simulink model "humanoidRobotIcub"  (Simulink 9.2)
settings: Solver=FixedStepAuto  StartTime=0.0  StopTime=10.0  FixedStep=0.001  RelTol=1e-3
undefined symbols (not defined in the file): DESIRED_TRAJECTORY_IS_FIXED, dq_max, dq_min, k1, k2, k3, q_des_amp, q_des_bias, q_des_freq, q_des_phase, q_max, q_min
libraries: WBToolboxLibrary x9
settings Model: Creator=venus.pasandi  LastModifiedBy=venus.pasandi
settings DataIOCC: LimitDataPoints=off  SaveFormat=Dataset  SignalLoggingSaveFormat=Dataset
settings OptimizationCC: LifeSpan=auto
settings DebuggingCC: UnderspecifiedInitializationDetection=Simplified  MergeDetectMultiDrivingBlocksExec=error  FcnCallInpInsideContextMsg=error  StateNameClashWarn=none  SFUnexpectedBacktrackingDiag=error  SFNoUnconditionalDefaultTransitionDiag=error  SFExecutionAtInitializationDiag=warning
settings HardwareCC: ProdBitPerPointer=64  ProdBitPerSizeT=64  ProdBitPerPtrDiffT=64  ProdLargestAtomicFloat=Float  ProdIntDivRoundTo=Zero  ProdEndianess=LittleEndian  ProdWordSize=64  ProdHWDeviceType=Intel->x86-64 (Windows64)
settings ModelReferenceCC: PropagateSignalLabelsOutOfModel=on
settings SFSimCC: SimUseLocalCustomCode=on
settings RTWCC: RTWUseLocalCustomCode=on
settings CodeAppCC: StateflowObjectComments=off
settings GRTTargetCC: TargetLangStandard=C99 (ISO)  GeneratePreprocessorConditionals=Use local settings  CombineOutputUpdateFcns=on  GRTInterface=off
settings ConfigComp: CovMetricSettings=dwe  CovHtmlReporting=off  CovSaveCumulativeToWorkspaceVar=off  CovSaveSingleToWorkspaceVar=off  CovExternalEMLEnable=on

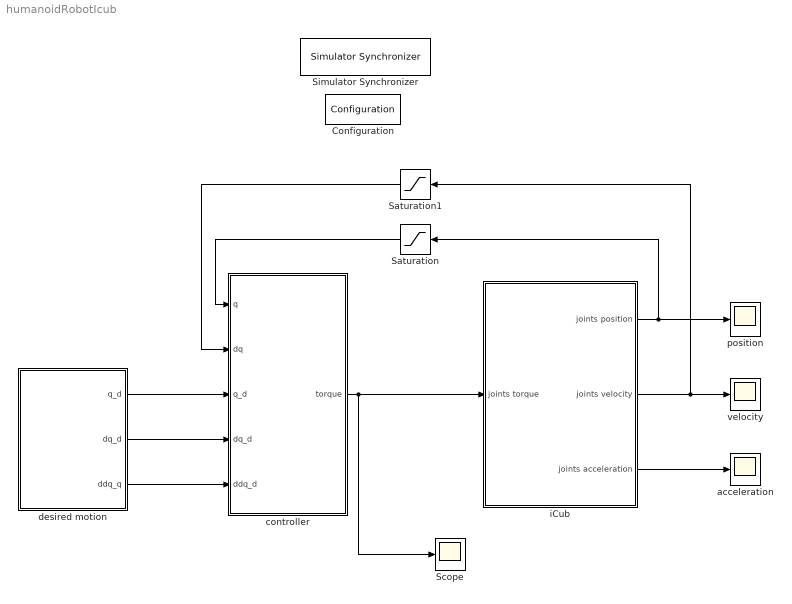
== system humanoidRobotIcub ==
  Configuration : WBToolboxLibrary/Utilities/Configuration  ConfigSource=Mask  ConfigObject='WBTConfigRobot'  RobotName='icubSim'  UrdfFile='model.urdf'  ControlledJoints={'r_hip_pitch', 'r_hip_roll', 'r_knee'}  ControlBoardsNames={'right_leg'}  LocalName='WBT'  GravityVector=[0,0,-9.81]
      settings: SourceProductName=WholeBodyToolbox
  Saturation : Saturate  UpperLimit=q_max-0.001  LowerLimit=q_min+0.001
  Saturation1 : Saturate  UpperLimit=dq_max-0.001  LowerLimit=dq_min+0.001
  Scope : Scope
  Simulator Synchronizer : WBToolboxLibrary/Utilities/Simulator Synchronizer  period=0.001  serverPortName='/clock/rpc'  clientPortName='/WBT_synchronizer/rpc:o'
      settings: SourceProductName=WholeBodyToolbox
  acceleration : Scope
  controller : Subsystem
  desired motion : Subsystem
  iCub : Subsystem
  position : Scope
  velocity : Scope
  wires:
  iCub/1(joints position) -> Saturation/1, position/1
  iCub/2(joints velocity) -> Saturation1/1, velocity/1
  iCub/3(joints acceleration) -> acceleration/1
  controller/1(torque) -> Scope/1, iCub/1(joints torque)
  desired motion/1(q_d) -> controller/3(q_d)
  desired motion/2(dq_d) -> controller/4(dq_d)
  desired motion/3(ddq_q) -> controller/5(ddq_d)
  Saturation/1 -> controller/1(q)
  Saturation1/1 -> controller/2(dq)

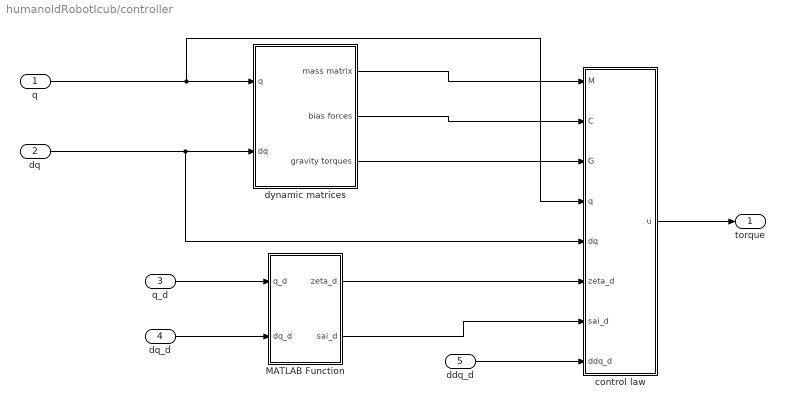
== system humanoidRobotIcub/controller ==
  q : Inport
  dq : Inport  Port=2
  q_d : Inport  Port=3
  dq_d : Inport  Port=4
  ddq_d : Inport  Port=5
  MATLAB Function : MATLAB Function  TreatAsAtomicUnit=on
  control law : MATLAB Function  TreatAsAtomicUnit=on
  dynamic matrices : Subsystem
  torque : Outport  VectorParamsAs1DForOutWhenUnconnected=on
  wires:
  dq_d/1 -> MATLAB Function/2(dq_d)
  q_d/1 -> MATLAB Function/1(q_d)
  MATLAB Function/2(sai_d) -> control law/7(sai_d)
  MATLAB Function/1(zeta_d) -> control law/6(zeta_d)
  control law/1(u) -> torque/1
  ddq_d/1 -> control law/8(ddq_d)
  dynamic matrices/3(gravity torques) -> control law/3(G)
  dynamic matrices/2(bias forces) -> control law/2(C)
  dynamic matrices/1(mass matrix) -> control law/1(M)
  dq/1 -> dynamic matrices/2(dq), control law/5(dq)
  q/1 -> control law/4(q), dynamic matrices/1(q)

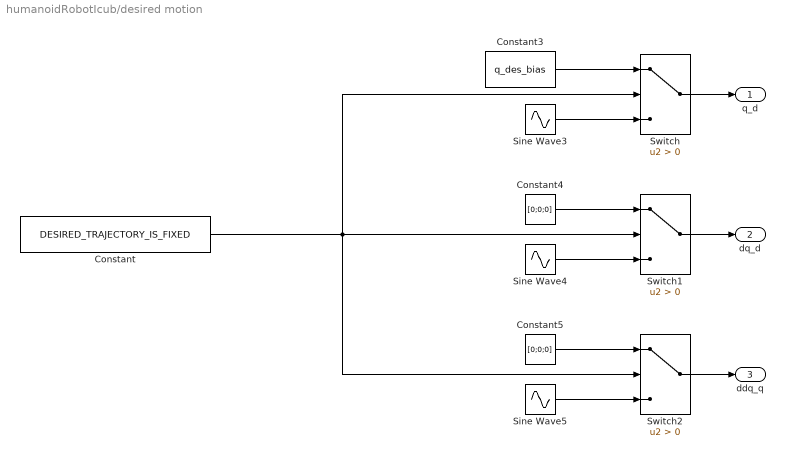
== system humanoidRobotIcub/desired motion ==
  Constant : Constant  Value=DESIRED_TRAJECTORY_IS_FIXED
  Constant3 : Constant  Value=q_des_bias
  Constant4 : Constant  Value=[0;0;0]
  Constant5 : Constant  Value=[0;0;0]
  Sine Wave3 : Sin  Amplitude=q_des_amp  Bias=q_des_bias  Frequency=q_des_freq  Phase=q_des_phase  SampleTime=0
  Sine Wave4 : Sin  Amplitude=q_des_amp .* q_des_freq  Bias=[0;0;0]  Frequency=q_des_freq  Phase=q_des_phase+pi/2  SampleTime=0
  Sine Wave5 : Sin  Amplitude=-q_des_amp .* (q_des_freq .^ 2)  Bias=[0;0;0]  Frequency=q_des_freq  Phase=q_des_phase  SampleTime=0
  Switch : Switch  Criteria=u2 > Threshold
  Switch1 : Switch  Criteria=u2 > Threshold
  Switch2 : Switch  Criteria=u2 > Threshold
  q_d : Outport  VectorParamsAs1DForOutWhenUnconnected=on
  dq_d : Outport  Port=2  VectorParamsAs1DForOutWhenUnconnected=on
  ddq_q : Outport  Port=3  VectorParamsAs1DForOutWhenUnconnected=on
  wires:
  Sine Wave5/1 -> Switch2/3
  Constant5/1 -> Switch2/1
  Constant4/1 -> Switch1/1
  Sine Wave4/1 -> Switch1/3
  Sine Wave3/1 -> Switch/3
  Constant3/1 -> Switch/1
  Constant/1 -> Switch/2, Switch2/2, Switch1/2
  Switch2/1 -> ddq_q/1
  Switch1/1 -> dq_d/1
  Switch/1 -> q_d/1

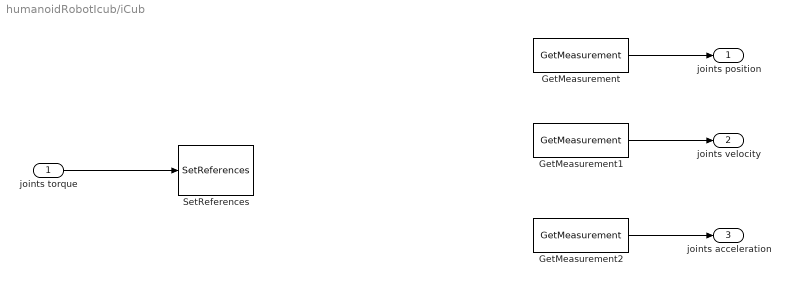
== system humanoidRobotIcub/iCub ==
  joints torque : Inport
  GetMeasurement : WBToolboxLibrary/States/GetMeasurement  measuredType=Joints Position
      settings: SourceProductName=WholeBodyToolbox
  GetMeasurement1 : WBToolboxLibrary/States/GetMeasurement  measuredType=Joints Velocity
      settings: SourceProductName=WholeBodyToolbox
  GetMeasurement2 : WBToolboxLibrary/States/GetMeasurement  measuredType=Joints Acceleration
      settings: SourceProductName=WholeBodyToolbox
  SetReferences : WBToolboxLibrary/Actuators/SetReferences  controlType=Torque  refSpeed=10*(pi/180)  refAcceleration=1000000*(pi/180)
      settings: SourceProductName=WholeBodyToolbox
  joints position : Outport
  joints velocity : Outport  Port=2
  joints acceleration : Outport  Port=3
  wires:
  GetMeasurement/1 -> joints position/1
  GetMeasurement1/1 -> joints velocity/1
  GetMeasurement2/1 -> joints acceleration/1
  joints torque/1 -> SetReferences/1

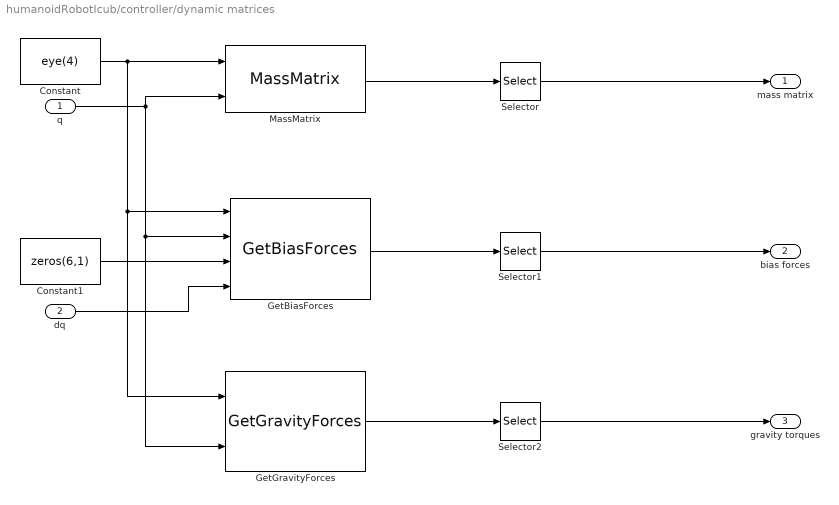
== system humanoidRobotIcub/controller/dynamic matrices ==
  q : Inport
  dq : Inport  Port=2
  Constant : Constant  Value=eye(4)
  Constant1 : Constant  Value=zeros(6,1)
  GetBiasForces : WBToolboxLibrary/Model/Dynamics/GetBiasForces
      settings: SourceProductName=WholeBodyToolbox
  GetGravityForces : WBToolboxLibrary/Model/Dynamics/GetGravityForces
      settings: SourceProductName=WholeBodyToolbox
  MassMatrix : WBToolboxLibrary/Model/Dynamics/MassMatrix
      settings: SourceProductName=WholeBodyToolbox
  Selector : Selector  NumberOfDimensions=2  InputPortWidth=3  IndexOptions=Index vector (dialog),Index vector (dialog)  Indices=[7:9],[7:9]  OutputSizes=1,1
  Selector1 : Selector  InputPortWidth=9  IndexOptions=Index vector (dialog)  Indices=[7:9]  OutputSizes=1
  Selector2 : Selector  InputPortWidth=9  IndexOptions=Index vector (dialog)  Indices=[7:9]  OutputSizes=1
  mass matrix : Outport
  bias forces : Outport  Port=2
  gravity torques : Outport  Port=3
  wires:
  Selector2/1 -> gravity torques/1
  Selector1/1 -> bias forces/1
  Selector/1 -> mass matrix/1
  dq/1 -> GetBiasForces/4
  Constant1/1 -> GetBiasForces/3
  GetBiasForces/1 -> Selector1/1
  GetGravityForces/1 -> Selector2/1
  MassMatrix/1 -> Selector/1
  q/1 -> MassMatrix/2, GetBiasForces/2, GetGravityForces/2
  Constant/1 -> MassMatrix/1, GetGravityForces/1, GetBiasForces/1

== matlab function controller/control law ==
  data: M input double; C input double; G input double; q input double; u output double; dq input double; zeta_d input double; sai_d input double; ddq_d input double; q_min parameter double; q_max parameter double; dq_min parameter double; dq_max parameter double; k1 parameter double; k2 parameter double; k3 parameter double
function u = fcn(M,C,G,q,dq,zeta_d,sai_d,ddq_d, q_min, q_max, dq_min, dq_max, k1, k2, k3)

%%%%%%%%%%%%%%%%%%%%%%%%%%%%%%%%%%%%%%%%%%%%%%%%%%%%%%%%%%%%%%%%%%%%%%%%%

q_avg = (q_max+q_min)/2;
dq_avg = (dq_max+dq_min)/2;

delta_q = diag((q_max-q_min)/2);
delta_dq = diag((dq_max-dq_min)/2);

%%%%%%%%%%%%%%%%%%%%%%%%%%%%%%%%%%%%%%%%%%%%%%%%%%%%%%%%%%%%%%%%%%%%%%%%%

zeta = atanh(delta_q\(q-q_avg));
sai = atanh(delta_dq\(dq-dq_avg));

%%%%%%%%%%%%%%%%%%%%%%%%%%%%%%%%%%%%%%%%%%%%%%%%%%%%%%%%%%%%%%%%%%%%%%%%%

J_zeta = delta_q*(eye(3)-diag(tanh(zeta))^2);
J_zeta_d = delta_q*(eye(3)-diag(tanh(zeta_d))^2);

J_sai = delta_dq*(eye(3)-diag(tanh(sai))^2);
J_sai_d = delta_dq*(eye(3)-diag(tanh(sai_d))^2);

%%%%%%%%%%%%%%%%%%%%%%%%%%%%%%%%%%%%%%%%%%%%%%%%%%%%%%%%%%%%%%%%%%%%%%%%%

dzeta = J_zeta\(dq_avg + delta_dq*tanh(sai));
dzeta_d = J_zeta_d\(dq_avg + delta_dq*tanh(sai_d));

dJ_zeta = -2*diag(tanh(zeta))*J_zeta*diag(dzeta);
dJ_zeta_d = -2*diag(tanh(zeta_d))*J_zeta_d*diag(dzeta_d);

dsai_d = J_sai_d\ddq_d;

%%%%%%%%%%%%%%%%%%%%%%%%%%%%%%%%%%%%%%%%%%%%%%%%%%%%%%%%%%%%%%%%%%%%%%%%%

p = 15;

tanh_bsai_r = delta_dq\(J_zeta/J_zeta_d*(dq_avg+delta_dq*tanh(sai_d)) - dq_avg);
sai_r =  atanh(tanh_bsai_r./(1+abs(tanh_bsai_r).^p).^(1/p));

J_sai_r = delta_dq*(eye(3)-diag(tanh(sai_r))^2);

dsai_r = J_sai_r\(dJ_zeta/J_zeta_d*(dq_avg+delta_dq*tanh(sai_d)) ...
    -J_zeta/J_zeta_d*dJ_zeta_d/J_zeta_d*(dq_avg+delta_dq*tanh(sai_d)) ...
    +J_zeta/J_zeta_d*delta_dq*(eye(3)-diag(tanh(sai_d))^2)*dsai_d);

%%%%%%%%%%%%%%%%%%%%%%%%%%%%%%%%%%%%%%%%%%%%%%%%%%%%%%%%%%%%%%%%%%%%%%%%%

e_zeta = zeta-zeta_d;
e_sai = sai-sai_r;

%%%%%%%%%%%%%%%%%%%%%%%%%%%%%%%%%%%%%%%%%%%%%%%%%%%%%%%%%%%%%%%%%%%%%%%%%

u = G + C + M*J_sai*(dsai_r - k2\k1/J_zeta*delta_dq ...
    *(tanh(sai)-tanh(sai_r)) - k2*e_zeta - k3/J_sai*e_sai);

== matlab function controller/MATLAB Function ==
  data: q_d input double; zeta_d output double; dq_d input double; sai_d output double; q_min parameter double; q_max parameter double; dq_min parameter double; dq_max parameter double
function [zeta_d,sai_d] = fcn(q_d,dq_d, q_min, q_max, dq_min, dq_max)

q_avg = (q_max+q_min)/2;
dq_avg = (dq_max+dq_min)/2;

delta_q = diag((q_max-q_min)/2);
delta_dq = diag((dq_max-dq_min)/2);

%%%%%%%%%%%%%%%%%%%%%%%%%%%%%%%%%%%%%%%%%%%%%%%%%%%%%%%%%%%%%%%%%%%%%%%%%

zeta_d = atanh(delta_q\(q_d-q_avg));
sai_d = atanh(delta_dq\(dq_d-dq_avg));
